simulink subsystem "Find_Catmull_Rom_Acc"  (R2023b)
settings: Solver=VariableStepAuto  StartTime=0.0  StopTime=10.0  RelTol=1e-3
settings Model: Creator=FIRSTMentor  LastModifiedBy=FIRSTMentor

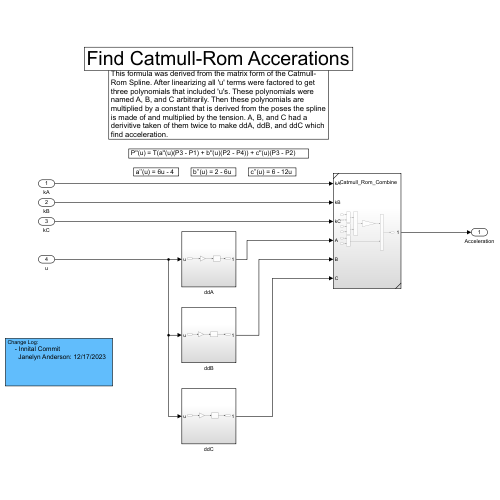
[thumbnail: Simulink's stored preview of the top-level diagram]
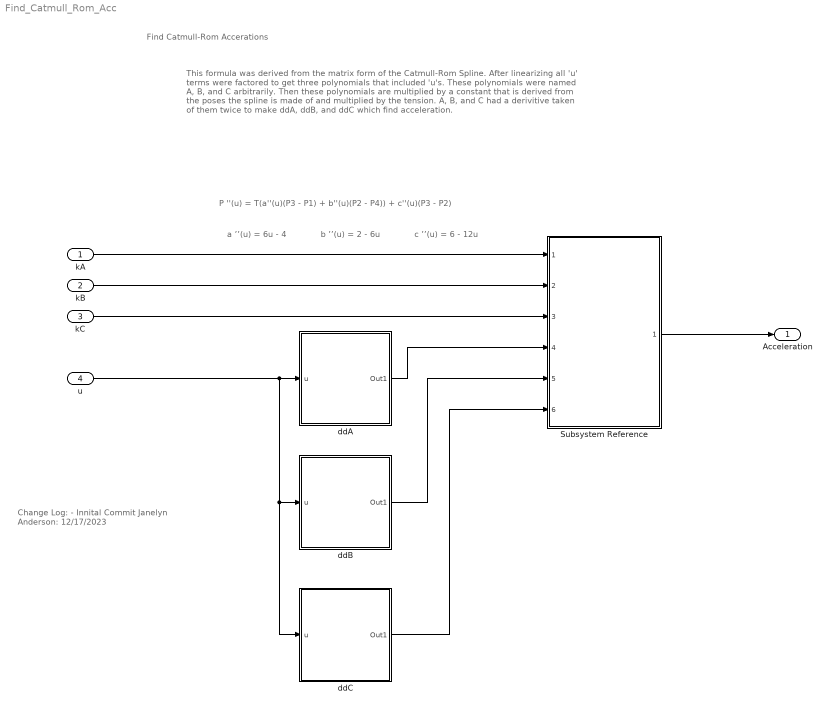
== system Find_Catmull_Rom_Acc ==
  note: a ’’(u) = 6u - 4
  note: P ''(u) = T(a''(u)(P3 - P1) + b''(u)(P2 - P4)) + c''(u)(P3 - P2)
  note: Change Log:
      | - Innital Commit
      | Janelyn Anderson: 12/17/2023
  note: Find Catmull-Rom Accerations
  note: This formula was derived from the matrix form of the Catmull-Rom Spline. After linearizing all 'u' terms were factored to get three polynomials that included 'u's. These polynomials were named A, B, and C arbitrarily. Then these polynomials are multiplied by a constant that is derived from the poses the spline is made of and multiplied by the tension. A, B, and C had a derivitive taken of them twice to make ddA, ddB, and ddC which find acceleration.
  note: b ’’(u) = 2 - 6u
  note: c ’’(u) = 6 - 12u
  kA : Inport  PortDimensions=[1 2]
  kB : Inport  Port=2  PortDimensions=[1 2]
  kC : Inport  Port=3  PortDimensions=[1 2]
  u : Inport  Port=4  PortDimensions=1
  Subsystem Reference : Subsystem  ReferencedSubsystem=Catmull_Rom_Combine
  ddA : Subsystem
  ddB : Subsystem
  ddC : Subsystem
  Acceleration : Outport
  wires:
  u/1 -> ddA/1(u), ddC/1(u), ddB/1(u)
  ddA/1(Out1) -> Subsystem Reference/4
  Subsystem Reference/1 -> Acceleration/1
  ddC/1(Out1) -> Subsystem Reference/6
  ddB/1(Out1) -> Subsystem Reference/5
  kB/1 -> Subsystem Reference/2
  kA/1 -> Subsystem Reference/1
  kC/1 -> Subsystem Reference/3

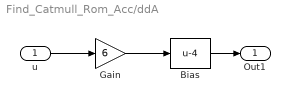
== system Find_Catmull_Rom_Acc/ddA ==
  u : Inport
  Bias : Bias  Bias=-4  SaturateOnIntegerOverflow=off
  Gain : Gain  Gain=6
  Out1 : Outport
  wires:
  Gain/1 -> Bias/1
  u/1 -> Gain/1
  Bias/1 -> Out1/1

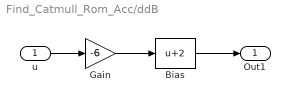
== system Find_Catmull_Rom_Acc/ddB ==
  u : Inport
  Bias : Bias  Bias=2  SaturateOnIntegerOverflow=off
  Gain : Gain  Gain=-6
  Out1 : Outport
  wires:
  Bias/1 -> Out1/1
  Gain/1 -> Bias/1
  u/1 -> Gain/1

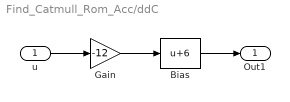
== system Find_Catmull_Rom_Acc/ddC ==
  u : Inport
  Bias : Bias  Bias=6  SaturateOnIntegerOverflow=off
  Gain : Gain  Gain=-12
  Out1 : Outport
  wires:
  Bias/1 -> Out1/1
  Gain/1 -> Bias/1
  u/1 -> Gain/1
